simulink model "model_cnn"  (R2020a)
settings: Solver=VariableStepAuto  StartTime=0.0  StopTime=1e6/fs  RelTol=1e-3
PreLoadFcn:
  | setup_imports;
  | %dense2_numerictype = fixdt(1,18,10);
  | %conv1_numerictype = fixdt(1,18,21);
InitFcn:
  | % Intermediate signal dimensions
  | input_dim = [1, 2, 128];
  | layer1_dim = hInterConvLayerDims([1,3,1,64],input_dim,1); % dims : [C,H,W]
  | layer2_dim = hInterConvLayerDims([2,3,64,16],layer1_dim,1);% dims : [C,H,W]
  | layer3_dim = [1,128];
  | 
  | % Conv Layer 1 dimensions
  | conv1_dims = struct(...
  |     'input_dim',    input_dim,...       input_dim = C,H,W
  |     'filter_dim',   [1, 3, 1, 64],...  filter_dim = K,J,C,N
  |     'stride',       1,...
  |     'row_output',   3,...
  |     'output_dim',   layer1_dim);
  | 
  | % Conv Layer 2 dimensions
  | conv2_dims = struct(...
  |     'input_dim',    layer1_dim,...      input = C,H.W
  |     'filter_dim',   [2, 3, 64, 16],...  filter_dim = K,J,C,N
  |     'stride',       1,...
  |     'row_output',   2*3*64,...
  |     'output_dim',   layer2_dim);
  | 
  | % Dense Layer 1 dimensions
  | dense1_dims = struct(...
  |     'input_dim',    layer2_dim,...      input = C,H,W
  |     'weight_dim',   [1984, 128],...     weight_dim = H,W
  |     'output_dim',   layer3_dim);
  | 
  | % Load saved weights and input
  | setup_imports;
  | 
  | fs = 128e6;
  | fs_axi = 100e6;
  | R = 32;
values from neighbouring files (symbols this model uses):
  datatypeInput = X_test.numerictype    [setup_imports.m]
  gemm_wconv1 = fi(hInterleaveFilters(Wconv1),1,16)    [setup_imports.m]
  gemm_wconv2 = fi(hInterleaveFilters(Wconv2),1,16)    [setup_imports.m]
  wdense1 = fi(Wdense1,1,16)    [setup_imports.m]
  wdense2 = fi(Wdense2,1,16)    [setup_imports.m]
undefined symbols (not defined in the file or in its folder): ltehdlRAMinitPO2
libraries: hdlsllib x1022, dspsigops x3, dspsrcs4 x2
(part 11 of 23)

== system model_cnn/HDL CNN Model/Dense Layer 1/Dense Layer 1/adder50 ==
  In1 : Inport
  In2 : Inport  Port=2
  In3 : Inport  Port=3
  Data Type Conversion : DataTypeConversion  OutDataTypeStr=datatypeLayer3
  Multiply-Accumulate : hdlsllib/HDL Operations/Multiply-Accumulate  opMode=Streaming - using Number of Samples  initValueSetting=Dialog  initValue=0  initValueSetting2=Dialog  initValue2=0  initValueSetting3=Dialog  initValue3=0  num_samples=1984  RndMeth2=Floor  RndMeth3=Floor  datatype2=Inherit: Inherit via back propagation  datatype3=accumoutdatatype3  validOut=on  endInandOut=on  startOut=on  countOut=on  dim=-1  DoSatur=off  parallel=off
      settings: SourceProductBaseCode=SL
  Terminator : Terminator
  Terminator1 : Terminator
  Terminator2 : Terminator
  dataOut : Outport
  wires:
  Data Type Conversion/1 -> dataOut/1
  ? -> Terminator1/1  "validOut"
  In2/1 -> Multiply-Accumulate/1
  In3/1 -> ?
  Multiply-Accumulate/1 -> Data Type Conversion/1
  ? -> Terminator/1  "countOut"
  In1/1 -> Multiply-Accumulate/2
  ? -> Terminator2/1  "vectorOutValid"

== system model_cnn/HDL CNN Model/Dense Layer 1/Dense Layer 1/adder51 ==
  In1 : Inport
  In2 : Inport  Port=2
  In3 : Inport  Port=3
  Data Type Conversion : DataTypeConversion  OutDataTypeStr=datatypeLayer3
  Multiply-Accumulate : hdlsllib/HDL Operations/Multiply-Accumulate  opMode=Streaming - using Number of Samples  initValueSetting=Dialog  initValue=0  initValueSetting2=Dialog  initValue2=0  initValueSetting3=Dialog  initValue3=0  num_samples=1984  RndMeth2=Floor  RndMeth3=Floor  datatype2=Inherit: Inherit via back propagation  datatype3=accumoutdatatype3  validOut=on  endInandOut=on  startOut=on  countOut=on  dim=-1  DoSatur=off  parallel=off
      settings: SourceProductBaseCode=SL
  Terminator : Terminator
  Terminator1 : Terminator
  Terminator2 : Terminator
  dataOut : Outport
  wires:
  Data Type Conversion/1 -> dataOut/1
  ? -> Terminator1/1  "validOut"
  In2/1 -> Multiply-Accumulate/1
  In3/1 -> ?
  Multiply-Accumulate/1 -> Data Type Conversion/1
  ? -> Terminator/1  "countOut"
  In1/1 -> Multiply-Accumulate/2
  ? -> Terminator2/1  "vectorOutValid"

== system model_cnn/HDL CNN Model/Dense Layer 1/Dense Layer 1/adder52 ==
  In1 : Inport
  In2 : Inport  Port=2
  In3 : Inport  Port=3
  Data Type Conversion : DataTypeConversion  OutDataTypeStr=datatypeLayer3
  Multiply-Accumulate : hdlsllib/HDL Operations/Multiply-Accumulate  opMode=Streaming - using Number of Samples  initValueSetting=Dialog  initValue=0  initValueSetting2=Dialog  initValue2=0  initValueSetting3=Dialog  initValue3=0  num_samples=1984  RndMeth2=Floor  RndMeth3=Floor  datatype2=Inherit: Inherit via back propagation  datatype3=accumoutdatatype3  validOut=on  endInandOut=on  startOut=on  countOut=on  dim=-1  DoSatur=off  parallel=off
      settings: SourceProductBaseCode=SL
  Terminator : Terminator
  Terminator1 : Terminator
  Terminator2 : Terminator
  dataOut : Outport
  wires:
  Data Type Conversion/1 -> dataOut/1
  ? -> Terminator1/1  "validOut"
  In2/1 -> Multiply-Accumulate/1
  In3/1 -> ?
  Multiply-Accumulate/1 -> Data Type Conversion/1
  ? -> Terminator/1  "countOut"
  In1/1 -> Multiply-Accumulate/2
  ? -> Terminator2/1  "vectorOutValid"

== system model_cnn/HDL CNN Model/Dense Layer 1/Dense Layer 1/adder53 ==
  In1 : Inport
  In2 : Inport  Port=2
  In3 : Inport  Port=3
  Data Type Conversion : DataTypeConversion  OutDataTypeStr=datatypeLayer3
  Multiply-Accumulate : hdlsllib/HDL Operations/Multiply-Accumulate  opMode=Streaming - using Number of Samples  initValueSetting=Dialog  initValue=0  initValueSetting2=Dialog  initValue2=0  initValueSetting3=Dialog  initValue3=0  num_samples=1984  RndMeth2=Floor  RndMeth3=Floor  datatype2=Inherit: Inherit via back propagation  datatype3=accumoutdatatype3  validOut=on  endInandOut=on  startOut=on  countOut=on  dim=-1  DoSatur=off  parallel=off
      settings: SourceProductBaseCode=SL
  Terminator : Terminator
  Terminator1 : Terminator
  Terminator2 : Terminator
  dataOut : Outport
  wires:
  Data Type Conversion/1 -> dataOut/1
  ? -> Terminator1/1  "validOut"
  In2/1 -> Multiply-Accumulate/1
  In3/1 -> ?
  Multiply-Accumulate/1 -> Data Type Conversion/1
  ? -> Terminator/1  "countOut"
  In1/1 -> Multiply-Accumulate/2
  ? -> Terminator2/1  "vectorOutValid"

== system model_cnn/HDL CNN Model/Dense Layer 1/Dense Layer 1/adder54 ==
  In1 : Inport
  In2 : Inport  Port=2
  In3 : Inport  Port=3
  Data Type Conversion : DataTypeConversion  OutDataTypeStr=datatypeLayer3
  Multiply-Accumulate : hdlsllib/HDL Operations/Multiply-Accumulate  opMode=Streaming - using Number of Samples  initValueSetting=Dialog  initValue=0  initValueSetting2=Dialog  initValue2=0  initValueSetting3=Dialog  initValue3=0  num_samples=1984  RndMeth2=Floor  RndMeth3=Floor  datatype2=Inherit: Inherit via back propagation  datatype3=accumoutdatatype3  validOut=on  endInandOut=on  startOut=on  countOut=on  dim=-1  DoSatur=off  parallel=off
      settings: SourceProductBaseCode=SL
  Terminator : Terminator
  Terminator1 : Terminator
  Terminator2 : Terminator
  dataOut : Outport
  wires:
  Data Type Conversion/1 -> dataOut/1
  ? -> Terminator1/1  "validOut"
  In2/1 -> Multiply-Accumulate/1
  In3/1 -> ?
  Multiply-Accumulate/1 -> Data Type Conversion/1
  ? -> Terminator/1  "countOut"
  In1/1 -> Multiply-Accumulate/2
  ? -> Terminator2/1  "vectorOutValid"

== system model_cnn/HDL CNN Model/Dense Layer 1/Dense Layer 1/adder55 ==
  In1 : Inport
  In2 : Inport  Port=2
  In3 : Inport  Port=3
  Data Type Conversion : DataTypeConversion  OutDataTypeStr=datatypeLayer3
  Multiply-Accumulate : hdlsllib/HDL Operations/Multiply-Accumulate  opMode=Streaming - using Number of Samples  initValueSetting=Dialog  initValue=0  initValueSetting2=Dialog  initValue2=0  initValueSetting3=Dialog  initValue3=0  num_samples=1984  RndMeth2=Floor  RndMeth3=Floor  datatype2=Inherit: Inherit via back propagation  datatype3=accumoutdatatype3  validOut=on  endInandOut=on  startOut=on  countOut=on  dim=-1  DoSatur=off  parallel=off
      settings: SourceProductBaseCode=SL
  Terminator : Terminator
  Terminator1 : Terminator
  Terminator2 : Terminator
  dataOut : Outport
  wires:
  Data Type Conversion/1 -> dataOut/1
  ? -> Terminator1/1  "validOut"
  In2/1 -> Multiply-Accumulate/1
  In3/1 -> ?
  Multiply-Accumulate/1 -> Data Type Conversion/1
  ? -> Terminator/1  "countOut"
  In1/1 -> Multiply-Accumulate/2
  ? -> Terminator2/1  "vectorOutValid"

== system model_cnn/HDL CNN Model/Dense Layer 1/Dense Layer 1/adder56 ==
  In1 : Inport
  In2 : Inport  Port=2
  In3 : Inport  Port=3
  Data Type Conversion : DataTypeConversion  OutDataTypeStr=datatypeLayer3
  Multiply-Accumulate : hdlsllib/HDL Operations/Multiply-Accumulate  opMode=Streaming - using Number of Samples  initValueSetting=Dialog  initValue=0  initValueSetting2=Dialog  initValue2=0  initValueSetting3=Dialog  initValue3=0  num_samples=1984  RndMeth2=Floor  RndMeth3=Floor  datatype2=Inherit: Inherit via back propagation  datatype3=accumoutdatatype3  validOut=on  endInandOut=on  startOut=on  countOut=on  dim=-1  DoSatur=off  parallel=off
      settings: SourceProductBaseCode=SL
  Terminator : Terminator
  Terminator1 : Terminator
  Terminator2 : Terminator
  dataOut : Outport
  wires:
  Data Type Conversion/1 -> dataOut/1
  ? -> Terminator1/1  "validOut"
  In2/1 -> Multiply-Accumulate/1
  In3/1 -> ?
  Multiply-Accumulate/1 -> Data Type Conversion/1
  ? -> Terminator/1  "countOut"
  In1/1 -> Multiply-Accumulate/2
  ? -> Terminator2/1  "vectorOutValid"

== system model_cnn/HDL CNN Model/Dense Layer 1/Dense Layer 1/adder57 ==
  In1 : Inport
  In2 : Inport  Port=2
  In3 : Inport  Port=3
  Data Type Conversion : DataTypeConversion  OutDataTypeStr=datatypeLayer3
  Multiply-Accumulate : hdlsllib/HDL Operations/Multiply-Accumulate  opMode=Streaming - using Number of Samples  initValueSetting=Dialog  initValue=0  initValueSetting2=Dialog  initValue2=0  initValueSetting3=Dialog  initValue3=0  num_samples=1984  RndMeth2=Floor  RndMeth3=Floor  datatype2=Inherit: Inherit via back propagation  datatype3=accumoutdatatype3  validOut=on  endInandOut=on  startOut=on  countOut=on  dim=-1  DoSatur=off  parallel=off
      settings: SourceProductBaseCode=SL
  Terminator : Terminator
  Terminator1 : Terminator
  Terminator2 : Terminator
  dataOut : Outport
  wires:
  Data Type Conversion/1 -> dataOut/1
  ? -> Terminator1/1  "validOut"
  In2/1 -> Multiply-Accumulate/1
  In3/1 -> ?
  Multiply-Accumulate/1 -> Data Type Conversion/1
  ? -> Terminator/1  "countOut"
  In1/1 -> Multiply-Accumulate/2
  ? -> Terminator2/1  "vectorOutValid"

== system model_cnn/HDL CNN Model/Dense Layer 1/Dense Layer 1/adder58 ==
  In1 : Inport
  In2 : Inport  Port=2
  In3 : Inport  Port=3
  Data Type Conversion : DataTypeConversion  OutDataTypeStr=datatypeLayer3
  Multiply-Accumulate : hdlsllib/HDL Operations/Multiply-Accumulate  opMode=Streaming - using Number of Samples  initValueSetting=Dialog  initValue=0  initValueSetting2=Dialog  initValue2=0  initValueSetting3=Dialog  initValue3=0  num_samples=1984  RndMeth2=Floor  RndMeth3=Floor  datatype2=Inherit: Inherit via back propagation  datatype3=accumoutdatatype3  validOut=on  endInandOut=on  startOut=on  countOut=on  dim=-1  DoSatur=off  parallel=off
      settings: SourceProductBaseCode=SL
  Terminator : Terminator
  Terminator1 : Terminator
  Terminator2 : Terminator
  dataOut : Outport
  wires:
  Data Type Conversion/1 -> dataOut/1
  ? -> Terminator1/1  "validOut"
  In2/1 -> Multiply-Accumulate/1
  In3/1 -> ?
  Multiply-Accumulate/1 -> Data Type Conversion/1
  ? -> Terminator/1  "countOut"
  In1/1 -> Multiply-Accumulate/2
  ? -> Terminator2/1  "vectorOutValid"

== system model_cnn/HDL CNN Model/Dense Layer 1/Dense Layer 1/adder59 ==
  In1 : Inport
  In2 : Inport  Port=2
  In3 : Inport  Port=3
  Data Type Conversion : DataTypeConversion  OutDataTypeStr=datatypeLayer3
  Multiply-Accumulate : hdlsllib/HDL Operations/Multiply-Accumulate  opMode=Streaming - using Number of Samples  initValueSetting=Dialog  initValue=0  initValueSetting2=Dialog  initValue2=0  initValueSetting3=Dialog  initValue3=0  num_samples=1984  RndMeth2=Floor  RndMeth3=Floor  datatype2=Inherit: Inherit via back propagation  datatype3=accumoutdatatype3  validOut=on  endInandOut=on  startOut=on  countOut=on  dim=-1  DoSatur=off  parallel=off
      settings: SourceProductBaseCode=SL
  Terminator : Terminator
  Terminator1 : Terminator
  Terminator2 : Terminator
  dataOut : Outport
  wires:
  Data Type Conversion/1 -> dataOut/1
  ? -> Terminator1/1  "validOut"
  In2/1 -> Multiply-Accumulate/1
  In3/1 -> ?
  Multiply-Accumulate/1 -> Data Type Conversion/1
  ? -> Terminator/1  "countOut"
  In1/1 -> Multiply-Accumulate/2
  ? -> Terminator2/1  "vectorOutValid"

== system model_cnn/HDL CNN Model/Dense Layer 1/Dense Layer 1/adder6 ==
  In1 : Inport
  In2 : Inport  Port=2
  In3 : Inport  Port=3
  Data Type Conversion : DataTypeConversion  OutDataTypeStr=datatypeLayer3
  Multiply-Accumulate : hdlsllib/HDL Operations/Multiply-Accumulate  opMode=Streaming - using Number of Samples  initValueSetting=Dialog  initValue=0  initValueSetting2=Dialog  initValue2=0  initValueSetting3=Dialog  initValue3=0  num_samples=1984  RndMeth2=Floor  RndMeth3=Floor  datatype2=Inherit: Inherit via back propagation  datatype3=accumoutdatatype3  validOut=on  endInandOut=on  startOut=on  countOut=on  dim=-1  DoSatur=off  parallel=off
      settings: SourceProductBaseCode=SL
  Terminator : Terminator
  Terminator1 : Terminator
  Terminator2 : Terminator
  dataOut : Outport
  wires:
  Data Type Conversion/1 -> dataOut/1
  ? -> Terminator1/1  "validOut"
  In2/1 -> Multiply-Accumulate/1
  In3/1 -> ?
  Multiply-Accumulate/1 -> Data Type Conversion/1
  ? -> Terminator/1  "countOut"
  In1/1 -> Multiply-Accumulate/2
  ? -> Terminator2/1  "vectorOutValid"

== system model_cnn/HDL CNN Model/Dense Layer 1/Dense Layer 1/adder60 ==
  In1 : Inport
  In2 : Inport  Port=2
  In3 : Inport  Port=3
  Data Type Conversion : DataTypeConversion  OutDataTypeStr=datatypeLayer3
  Multiply-Accumulate : hdlsllib/HDL Operations/Multiply-Accumulate  opMode=Streaming - using Number of Samples  initValueSetting=Dialog  initValue=0  initValueSetting2=Dialog  initValue2=0  initValueSetting3=Dialog  initValue3=0  num_samples=1984  RndMeth2=Floor  RndMeth3=Floor  datatype2=Inherit: Inherit via back propagation  datatype3=accumoutdatatype3  validOut=on  endInandOut=on  startOut=on  countOut=on  dim=-1  DoSatur=off  parallel=off
      settings: SourceProductBaseCode=SL
  Terminator : Terminator
  Terminator1 : Terminator
  Terminator2 : Terminator
  dataOut : Outport
  wires:
  Data Type Conversion/1 -> dataOut/1
  ? -> Terminator1/1  "validOut"
  In2/1 -> Multiply-Accumulate/1
  In3/1 -> ?
  Multiply-Accumulate/1 -> Data Type Conversion/1
  ? -> Terminator/1  "countOut"
  In1/1 -> Multiply-Accumulate/2
  ? -> Terminator2/1  "vectorOutValid"

== system model_cnn/HDL CNN Model/Dense Layer 1/Dense Layer 1/adder61 ==
  In1 : Inport
  In2 : Inport  Port=2
  In3 : Inport  Port=3
  Data Type Conversion : DataTypeConversion  OutDataTypeStr=datatypeLayer3
  Multiply-Accumulate : hdlsllib/HDL Operations/Multiply-Accumulate  opMode=Streaming - using Number of Samples  initValueSetting=Dialog  initValue=0  initValueSetting2=Dialog  initValue2=0  initValueSetting3=Dialog  initValue3=0  num_samples=1984  RndMeth2=Floor  RndMeth3=Floor  datatype2=Inherit: Inherit via back propagation  datatype3=accumoutdatatype3  validOut=on  endInandOut=on  startOut=on  countOut=on  dim=-1  DoSatur=off  parallel=off
      settings: SourceProductBaseCode=SL
  Terminator : Terminator
  Terminator1 : Terminator
  Terminator2 : Terminator
  dataOut : Outport
  wires:
  Data Type Conversion/1 -> dataOut/1
  ? -> Terminator1/1  "validOut"
  In2/1 -> Multiply-Accumulate/1
  In3/1 -> ?
  Multiply-Accumulate/1 -> Data Type Conversion/1
  ? -> Terminator/1  "countOut"
  In1/1 -> Multiply-Accumulate/2
  ? -> Terminator2/1  "vectorOutValid"

== system model_cnn/HDL CNN Model/Dense Layer 1/Dense Layer 1/adder62 ==
  In1 : Inport
  In2 : Inport  Port=2
  In3 : Inport  Port=3
  Data Type Conversion : DataTypeConversion  OutDataTypeStr=datatypeLayer3
  Multiply-Accumulate : hdlsllib/HDL Operations/Multiply-Accumulate  opMode=Streaming - using Number of Samples  initValueSetting=Dialog  initValue=0  initValueSetting2=Dialog  initValue2=0  initValueSetting3=Dialog  initValue3=0  num_samples=1984  RndMeth2=Floor  RndMeth3=Floor  datatype2=Inherit: Inherit via back propagation  datatype3=accumoutdatatype3  validOut=on  endInandOut=on  startOut=on  countOut=on  dim=-1  DoSatur=off  parallel=off
      settings: SourceProductBaseCode=SL
  Terminator : Terminator
  Terminator1 : Terminator
  Terminator2 : Terminator
  dataOut : Outport
  wires:
  Data Type Conversion/1 -> dataOut/1
  ? -> Terminator1/1  "validOut"
  In2/1 -> Multiply-Accumulate/1
  In3/1 -> ?
  Multiply-Accumulate/1 -> Data Type Conversion/1
  ? -> Terminator/1  "countOut"
  In1/1 -> Multiply-Accumulate/2
  ? -> Terminator2/1  "vectorOutValid"

== system model_cnn/HDL CNN Model/Dense Layer 1/Dense Layer 1/adder63 ==
  In1 : Inport
  In2 : Inport  Port=2
  In3 : Inport  Port=3
  Data Type Conversion : DataTypeConversion  OutDataTypeStr=datatypeLayer3
  Multiply-Accumulate : hdlsllib/HDL Operations/Multiply-Accumulate  opMode=Streaming - using Number of Samples  initValueSetting=Dialog  initValue=0  initValueSetting2=Dialog  initValue2=0  initValueSetting3=Dialog  initValue3=0  num_samples=1984  RndMeth2=Floor  RndMeth3=Floor  datatype2=Inherit: Inherit via back propagation  datatype3=accumoutdatatype3  validOut=on  endInandOut=on  startOut=on  countOut=on  dim=-1  DoSatur=off  parallel=off
      settings: SourceProductBaseCode=SL
  Terminator : Terminator
  Terminator1 : Terminator
  Terminator2 : Terminator
  dataOut : Outport
  wires:
  Data Type Conversion/1 -> dataOut/1
  ? -> Terminator1/1  "validOut"
  In2/1 -> Multiply-Accumulate/1
  In3/1 -> ?
  Multiply-Accumulate/1 -> Data Type Conversion/1
  ? -> Terminator/1  "countOut"
  In1/1 -> Multiply-Accumulate/2
  ? -> Terminator2/1  "vectorOutValid"

== system model_cnn/HDL CNN Model/Dense Layer 1/Dense Layer 1/adder64 ==
  In1 : Inport
  In2 : Inport  Port=2
  In3 : Inport  Port=3
  Data Type Conversion : DataTypeConversion  OutDataTypeStr=datatypeLayer3
  Multiply-Accumulate : hdlsllib/HDL Operations/Multiply-Accumulate  opMode=Streaming - using Number of Samples  initValueSetting=Dialog  initValue=0  initValueSetting2=Dialog  initValue2=0  initValueSetting3=Dialog  initValue3=0  num_samples=1984  RndMeth2=Floor  RndMeth3=Floor  datatype2=Inherit: Inherit via back propagation  datatype3=accumoutdatatype3  validOut=on  endInandOut=on  startOut=on  countOut=on  dim=-1  DoSatur=off  parallel=off
      settings: SourceProductBaseCode=SL
  Terminator : Terminator
  Terminator1 : Terminator
  Terminator2 : Terminator
  dataOut : Outport
  wires:
  Data Type Conversion/1 -> dataOut/1
  ? -> Terminator1/1  "validOut"
  In2/1 -> Multiply-Accumulate/1
  In3/1 -> ?
  Multiply-Accumulate/1 -> Data Type Conversion/1
  ? -> Terminator/1  "countOut"
  In1/1 -> Multiply-Accumulate/2
  ? -> Terminator2/1  "vectorOutValid"

== system model_cnn/HDL CNN Model/Dense Layer 1/Dense Layer 1/adder65 ==
  In1 : Inport
  In2 : Inport  Port=2
  In3 : Inport  Port=3
  Data Type Conversion : DataTypeConversion  OutDataTypeStr=datatypeLayer3
  Multiply-Accumulate : hdlsllib/HDL Operations/Multiply-Accumulate  opMode=Streaming - using Number of Samples  initValueSetting=Dialog  initValue=0  initValueSetting2=Dialog  initValue2=0  initValueSetting3=Dialog  initValue3=0  num_samples=1984  RndMeth2=Floor  RndMeth3=Floor  datatype2=Inherit: Inherit via back propagation  datatype3=accumoutdatatype3  validOut=on  endInandOut=on  startOut=on  countOut=on  dim=-1  DoSatur=off  parallel=off
      settings: SourceProductBaseCode=SL
  Terminator : Terminator
  Terminator1 : Terminator
  Terminator2 : Terminator
  dataOut : Outport
  wires:
  Data Type Conversion/1 -> dataOut/1
  ? -> Terminator1/1  "validOut"
  In2/1 -> Multiply-Accumulate/1
  In3/1 -> ?
  Multiply-Accumulate/1 -> Data Type Conversion/1
  ? -> Terminator/1  "countOut"
  In1/1 -> Multiply-Accumulate/2
  ? -> Terminator2/1  "vectorOutValid"

== system model_cnn/HDL CNN Model/Dense Layer 1/Dense Layer 1/adder66 ==
  In1 : Inport
  In2 : Inport  Port=2
  In3 : Inport  Port=3
  Data Type Conversion : DataTypeConversion  OutDataTypeStr=datatypeLayer3
  Multiply-Accumulate : hdlsllib/HDL Operations/Multiply-Accumulate  opMode=Streaming - using Number of Samples  initValueSetting=Dialog  initValue=0  initValueSetting2=Dialog  initValue2=0  initValueSetting3=Dialog  initValue3=0  num_samples=1984  RndMeth2=Floor  RndMeth3=Floor  datatype2=Inherit: Inherit via back propagation  datatype3=accumoutdatatype3  validOut=on  endInandOut=on  startOut=on  countOut=on  dim=-1  DoSatur=off  parallel=off
      settings: SourceProductBaseCode=SL
  Terminator : Terminator
  Terminator1 : Terminator
  Terminator2 : Terminator
  dataOut : Outport
  wires:
  Data Type Conversion/1 -> dataOut/1
  ? -> Terminator1/1  "validOut"
  In2/1 -> Multiply-Accumulate/1
  In3/1 -> ?
  Multiply-Accumulate/1 -> Data Type Conversion/1
  ? -> Terminator/1  "countOut"
  In1/1 -> Multiply-Accumulate/2
  ? -> Terminator2/1  "vectorOutValid"

== system model_cnn/HDL CNN Model/Dense Layer 1/Dense Layer 1/adder67 ==
  In1 : Inport
  In2 : Inport  Port=2
  In3 : Inport  Port=3
  Data Type Conversion : DataTypeConversion  OutDataTypeStr=datatypeLayer3
  Multiply-Accumulate : hdlsllib/HDL Operations/Multiply-Accumulate  opMode=Streaming - using Number of Samples  initValueSetting=Dialog  initValue=0  initValueSetting2=Dialog  initValue2=0  initValueSetting3=Dialog  initValue3=0  num_samples=1984  RndMeth2=Floor  RndMeth3=Floor  datatype2=Inherit: Inherit via back propagation  datatype3=accumoutdatatype3  validOut=on  endInandOut=on  startOut=on  countOut=on  dim=-1  DoSatur=off  parallel=off
      settings: SourceProductBaseCode=SL
  Terminator : Terminator
  Terminator1 : Terminator
  Terminator2 : Terminator
  dataOut : Outport
  wires:
  Data Type Conversion/1 -> dataOut/1
  ? -> Terminator1/1  "validOut"
  In2/1 -> Multiply-Accumulate/1
  In3/1 -> ?
  Multiply-Accumulate/1 -> Data Type Conversion/1
  ? -> Terminator/1  "countOut"
  In1/1 -> Multiply-Accumulate/2
  ? -> Terminator2/1  "vectorOutValid"

== system model_cnn/HDL CNN Model/Dense Layer 1/Dense Layer 1/adder68 ==
  In1 : Inport
  In2 : Inport  Port=2
  In3 : Inport  Port=3
  Data Type Conversion : DataTypeConversion  OutDataTypeStr=datatypeLayer3
  Multiply-Accumulate : hdlsllib/HDL Operations/Multiply-Accumulate  opMode=Streaming - using Number of Samples  initValueSetting=Dialog  initValue=0  initValueSetting2=Dialog  initValue2=0  initValueSetting3=Dialog  initValue3=0  num_samples=1984  RndMeth2=Floor  RndMeth3=Floor  datatype2=Inherit: Inherit via back propagation  datatype3=accumoutdatatype3  validOut=on  endInandOut=on  startOut=on  countOut=on  dim=-1  DoSatur=off  parallel=off
      settings: SourceProductBaseCode=SL
  Terminator : Terminator
  Terminator1 : Terminator
  Terminator2 : Terminator
  dataOut : Outport
  wires:
  Data Type Conversion/1 -> dataOut/1
  ? -> Terminator1/1  "validOut"
  In2/1 -> Multiply-Accumulate/1
  In3/1 -> ?
  Multiply-Accumulate/1 -> Data Type Conversion/1
  ? -> Terminator/1  "countOut"
  In1/1 -> Multiply-Accumulate/2
  ? -> Terminator2/1  "vectorOutValid"

== system model_cnn/HDL CNN Model/Dense Layer 1/Dense Layer 1/adder69 ==
  In1 : Inport
  In2 : Inport  Port=2
  In3 : Inport  Port=3
  Data Type Conversion : DataTypeConversion  OutDataTypeStr=datatypeLayer3
  Multiply-Accumulate : hdlsllib/HDL Operations/Multiply-Accumulate  opMode=Streaming - using Number of Samples  initValueSetting=Dialog  initValue=0  initValueSetting2=Dialog  initValue2=0  initValueSetting3=Dialog  initValue3=0  num_samples=1984  RndMeth2=Floor  RndMeth3=Floor  datatype2=Inherit: Inherit via back propagation  datatype3=accumoutdatatype3  validOut=on  endInandOut=on  startOut=on  countOut=on  dim=-1  DoSatur=off  parallel=off
      settings: SourceProductBaseCode=SL
  Terminator : Terminator
  Terminator1 : Terminator
  Terminator2 : Terminator
  dataOut : Outport
  wires:
  Data Type Conversion/1 -> dataOut/1
  ? -> Terminator1/1  "validOut"
  In2/1 -> Multiply-Accumulate/1
  In3/1 -> ?
  Multiply-Accumulate/1 -> Data Type Conversion/1
  ? -> Terminator/1  "countOut"
  In1/1 -> Multiply-Accumulate/2
  ? -> Terminator2/1  "vectorOutValid"

== system model_cnn/HDL CNN Model/Dense Layer 1/Dense Layer 1/adder7 ==
  In1 : Inport
  In2 : Inport  Port=2
  In3 : Inport  Port=3
  Data Type Conversion : DataTypeConversion  OutDataTypeStr=datatypeLayer3
  Multiply-Accumulate : hdlsllib/HDL Operations/Multiply-Accumulate  opMode=Streaming - using Number of Samples  initValueSetting=Dialog  initValue=0  initValueSetting2=Dialog  initValue2=0  initValueSetting3=Dialog  initValue3=0  num_samples=1984  RndMeth2=Floor  RndMeth3=Floor  datatype2=Inherit: Inherit via back propagation  datatype3=accumoutdatatype3  validOut=on  endInandOut=on  startOut=on  countOut=on  dim=-1  DoSatur=off  parallel=off
      settings: SourceProductBaseCode=SL
  Terminator : Terminator
  Terminator1 : Terminator
  Terminator2 : Terminator
  dataOut : Outport
  wires:
  Data Type Conversion/1 -> dataOut/1
  ? -> Terminator1/1  "validOut"
  In2/1 -> Multiply-Accumulate/1
  In3/1 -> ?
  Multiply-Accumulate/1 -> Data Type Conversion/1
  ? -> Terminator/1  "countOut"
  In1/1 -> Multiply-Accumulate/2
  ? -> Terminator2/1  "vectorOutValid"

== system model_cnn/HDL CNN Model/Dense Layer 1/Dense Layer 1/adder70 ==
  In1 : Inport
  In2 : Inport  Port=2
  In3 : Inport  Port=3
  Data Type Conversion : DataTypeConversion  OutDataTypeStr=datatypeLayer3
  Multiply-Accumulate : hdlsllib/HDL Operations/Multiply-Accumulate  opMode=Streaming - using Number of Samples  initValueSetting=Dialog  initValue=0  initValueSetting2=Dialog  initValue2=0  initValueSetting3=Dialog  initValue3=0  num_samples=1984  RndMeth2=Floor  RndMeth3=Floor  datatype2=Inherit: Inherit via back propagation  datatype3=accumoutdatatype3  validOut=on  endInandOut=on  startOut=on  countOut=on  dim=-1  DoSatur=off  parallel=off
      settings: SourceProductBaseCode=SL
  Terminator : Terminator
  Terminator1 : Terminator
  Terminator2 : Terminator
  dataOut : Outport
  wires:
  Data Type Conversion/1 -> dataOut/1
  ? -> Terminator1/1  "validOut"
  In2/1 -> Multiply-Accumulate/1
  In3/1 -> ?
  Multiply-Accumulate/1 -> Data Type Conversion/1
  ? -> Terminator/1  "countOut"
  In1/1 -> Multiply-Accumulate/2
  ? -> Terminator2/1  "vectorOutValid"

== system model_cnn/HDL CNN Model/Dense Layer 1/Dense Layer 1/adder71 ==
  In1 : Inport
  In2 : Inport  Port=2
  In3 : Inport  Port=3
  Data Type Conversion : DataTypeConversion  OutDataTypeStr=datatypeLayer3
  Multiply-Accumulate : hdlsllib/HDL Operations/Multiply-Accumulate  opMode=Streaming - using Number of Samples  initValueSetting=Dialog  initValue=0  initValueSetting2=Dialog  initValue2=0  initValueSetting3=Dialog  initValue3=0  num_samples=1984  RndMeth2=Floor  RndMeth3=Floor  datatype2=Inherit: Inherit via back propagation  datatype3=accumoutdatatype3  validOut=on  endInandOut=on  startOut=on  countOut=on  dim=-1  DoSatur=off  parallel=off
      settings: SourceProductBaseCode=SL
  Terminator : Terminator
  Terminator1 : Terminator
  Terminator2 : Terminator
  dataOut : Outport
  wires:
  Data Type Conversion/1 -> dataOut/1
  ? -> Terminator1/1  "validOut"
  In2/1 -> Multiply-Accumulate/1
  In3/1 -> ?
  Multiply-Accumulate/1 -> Data Type Conversion/1
  ? -> Terminator/1  "countOut"
  In1/1 -> Multiply-Accumulate/2
  ? -> Terminator2/1  "vectorOutValid"

== system model_cnn/HDL CNN Model/Dense Layer 1/Dense Layer 1/adder72 ==
  In1 : Inport
  In2 : Inport  Port=2
  In3 : Inport  Port=3
  Data Type Conversion : DataTypeConversion  OutDataTypeStr=datatypeLayer3
  Multiply-Accumulate : hdlsllib/HDL Operations/Multiply-Accumulate  opMode=Streaming - using Number of Samples  initValueSetting=Dialog  initValue=0  initValueSetting2=Dialog  initValue2=0  initValueSetting3=Dialog  initValue3=0  num_samples=1984  RndMeth2=Floor  RndMeth3=Floor  datatype2=Inherit: Inherit via back propagation  datatype3=accumoutdatatype3  validOut=on  endInandOut=on  startOut=on  countOut=on  dim=-1  DoSatur=off  parallel=off
      settings: SourceProductBaseCode=SL
  Terminator : Terminator
  Terminator1 : Terminator
  Terminator2 : Terminator
  dataOut : Outport
  wires:
  Data Type Conversion/1 -> dataOut/1
  ? -> Terminator1/1  "validOut"
  In2/1 -> Multiply-Accumulate/1
  In3/1 -> ?
  Multiply-Accumulate/1 -> Data Type Conversion/1
  ? -> Terminator/1  "countOut"
  In1/1 -> Multiply-Accumulate/2
  ? -> Terminator2/1  "vectorOutValid"

== system model_cnn/HDL CNN Model/Dense Layer 1/Dense Layer 1/adder73 ==
  In1 : Inport
  In2 : Inport  Port=2
  In3 : Inport  Port=3
  Data Type Conversion : DataTypeConversion  OutDataTypeStr=datatypeLayer3
  Multiply-Accumulate : hdlsllib/HDL Operations/Multiply-Accumulate  opMode=Streaming - using Number of Samples  initValueSetting=Dialog  initValue=0  initValueSetting2=Dialog  initValue2=0  initValueSetting3=Dialog  initValue3=0  num_samples=1984  RndMeth2=Floor  RndMeth3=Floor  datatype2=Inherit: Inherit via back propagation  datatype3=accumoutdatatype3  validOut=on  endInandOut=on  startOut=on  countOut=on  dim=-1  DoSatur=off  parallel=off
      settings: SourceProductBaseCode=SL
  Terminator : Terminator
  Terminator1 : Terminator
  Terminator2 : Terminator
  dataOut : Outport
  wires:
  Data Type Conversion/1 -> dataOut/1
  ? -> Terminator1/1  "validOut"
  In2/1 -> Multiply-Accumulate/1
  In3/1 -> ?
  Multiply-Accumulate/1 -> Data Type Conversion/1
  ? -> Terminator/1  "countOut"
  In1/1 -> Multiply-Accumulate/2
  ? -> Terminator2/1  "vectorOutValid"

== system model_cnn/HDL CNN Model/Dense Layer 1/Dense Layer 1/adder74 ==
  In1 : Inport
  In2 : Inport  Port=2
  In3 : Inport  Port=3
  Data Type Conversion : DataTypeConversion  OutDataTypeStr=datatypeLayer3
  Multiply-Accumulate : hdlsllib/HDL Operations/Multiply-Accumulate  opMode=Streaming - using Number of Samples  initValueSetting=Dialog  initValue=0  initValueSetting2=Dialog  initValue2=0  initValueSetting3=Dialog  initValue3=0  num_samples=1984  RndMeth2=Floor  RndMeth3=Floor  datatype2=Inherit: Inherit via back propagation  datatype3=accumoutdatatype3  validOut=on  endInandOut=on  startOut=on  countOut=on  dim=-1  DoSatur=off  parallel=off
      settings: SourceProductBaseCode=SL
  Terminator : Terminator
  Terminator1 : Terminator
  Terminator2 : Terminator
  dataOut : Outport
  wires:
  Data Type Conversion/1 -> dataOut/1
  ? -> Terminator1/1  "validOut"
  In2/1 -> Multiply-Accumulate/1
  In3/1 -> ?
  Multiply-Accumulate/1 -> Data Type Conversion/1
  ? -> Terminator/1  "countOut"
  In1/1 -> Multiply-Accumulate/2
  ? -> Terminator2/1  "vectorOutValid"

== system model_cnn/HDL CNN Model/Dense Layer 1/Dense Layer 1/adder75 ==
  In1 : Inport
  In2 : Inport  Port=2
  In3 : Inport  Port=3
  Data Type Conversion : DataTypeConversion  OutDataTypeStr=datatypeLayer3
  Multiply-Accumulate : hdlsllib/HDL Operations/Multiply-Accumulate  opMode=Streaming - using Number of Samples  initValueSetting=Dialog  initValue=0  initValueSetting2=Dialog  initValue2=0  initValueSetting3=Dialog  initValue3=0  num_samples=1984  RndMeth2=Floor  RndMeth3=Floor  datatype2=Inherit: Inherit via back propagation  datatype3=accumoutdatatype3  validOut=on  endInandOut=on  startOut=on  countOut=on  dim=-1  DoSatur=off  parallel=off
      settings: SourceProductBaseCode=SL
  Terminator : Terminator
  Terminator1 : Terminator
  Terminator2 : Terminator
  dataOut : Outport
  wires:
  Data Type Conversion/1 -> dataOut/1
  ? -> Terminator1/1  "validOut"
  In2/1 -> Multiply-Accumulate/1
  In3/1 -> ?
  Multiply-Accumulate/1 -> Data Type Conversion/1
  ? -> Terminator/1  "countOut"
  In1/1 -> Multiply-Accumulate/2
  ? -> Terminator2/1  "vectorOutValid"

== system model_cnn/HDL CNN Model/Dense Layer 1/Dense Layer 1/adder76 ==
  In1 : Inport
  In2 : Inport  Port=2
  In3 : Inport  Port=3
  Data Type Conversion : DataTypeConversion  OutDataTypeStr=datatypeLayer3
  Multiply-Accumulate : hdlsllib/HDL Operations/Multiply-Accumulate  opMode=Streaming - using Number of Samples  initValueSetting=Dialog  initValue=0  initValueSetting2=Dialog  initValue2=0  initValueSetting3=Dialog  initValue3=0  num_samples=1984  RndMeth2=Floor  RndMeth3=Floor  datatype2=Inherit: Inherit via back propagation  datatype3=accumoutdatatype3  validOut=on  endInandOut=on  startOut=on  countOut=on  dim=-1  DoSatur=off  parallel=off
      settings: SourceProductBaseCode=SL
  Terminator : Terminator
  Terminator1 : Terminator
  Terminator2 : Terminator
  dataOut : Outport
  wires:
  Data Type Conversion/1 -> dataOut/1
  ? -> Terminator1/1  "validOut"
  In2/1 -> Multiply-Accumulate/1
  In3/1 -> ?
  Multiply-Accumulate/1 -> Data Type Conversion/1
  ? -> Terminator/1  "countOut"
  In1/1 -> Multiply-Accumulate/2
  ? -> Terminator2/1  "vectorOutValid"

== system model_cnn/HDL CNN Model/Dense Layer 1/Dense Layer 1/adder77 ==
  In1 : Inport
  In2 : Inport  Port=2
  In3 : Inport  Port=3
  Data Type Conversion : DataTypeConversion  OutDataTypeStr=datatypeLayer3
  Multiply-Accumulate : hdlsllib/HDL Operations/Multiply-Accumulate  opMode=Streaming - using Number of Samples  initValueSetting=Dialog  initValue=0  initValueSetting2=Dialog  initValue2=0  initValueSetting3=Dialog  initValue3=0  num_samples=1984  RndMeth2=Floor  RndMeth3=Floor  datatype2=Inherit: Inherit via back propagation  datatype3=accumoutdatatype3  validOut=on  endInandOut=on  startOut=on  countOut=on  dim=-1  DoSatur=off  parallel=off
      settings: SourceProductBaseCode=SL
  Terminator : Terminator
  Terminator1 : Terminator
  Terminator2 : Terminator
  dataOut : Outport
  wires:
  Data Type Conversion/1 -> dataOut/1
  ? -> Terminator1/1  "validOut"
  In2/1 -> Multiply-Accumulate/1
  In3/1 -> ?
  Multiply-Accumulate/1 -> Data Type Conversion/1
  ? -> Terminator/1  "countOut"
  In1/1 -> Multiply-Accumulate/2
  ? -> Terminator2/1  "vectorOutValid"

== system model_cnn/HDL CNN Model/Dense Layer 1/Dense Layer 1/adder78 ==
  In1 : Inport
  In2 : Inport  Port=2
  In3 : Inport  Port=3
  Data Type Conversion : DataTypeConversion  OutDataTypeStr=datatypeLayer3
  Multiply-Accumulate : hdlsllib/HDL Operations/Multiply-Accumulate  opMode=Streaming - using Number of Samples  initValueSetting=Dialog  initValue=0  initValueSetting2=Dialog  initValue2=0  initValueSetting3=Dialog  initValue3=0  num_samples=1984  RndMeth2=Floor  RndMeth3=Floor  datatype2=Inherit: Inherit via back propagation  datatype3=accumoutdatatype3  validOut=on  endInandOut=on  startOut=on  countOut=on  dim=-1  DoSatur=off  parallel=off
      settings: SourceProductBaseCode=SL
  Terminator : Terminator
  Terminator1 : Terminator
  Terminator2 : Terminator
  dataOut : Outport
  wires:
  Data Type Conversion/1 -> dataOut/1
  ? -> Terminator1/1  "validOut"
  In2/1 -> Multiply-Accumulate/1
  In3/1 -> ?
  Multiply-Accumulate/1 -> Data Type Conversion/1
  ? -> Terminator/1  "countOut"
  In1/1 -> Multiply-Accumulate/2
  ? -> Terminator2/1  "vectorOutValid"

== system model_cnn/HDL CNN Model/Dense Layer 1/Dense Layer 1/adder79 ==
  In1 : Inport
  In2 : Inport  Port=2
  In3 : Inport  Port=3
  Data Type Conversion : DataTypeConversion  OutDataTypeStr=datatypeLayer3
  Multiply-Accumulate : hdlsllib/HDL Operations/Multiply-Accumulate  opMode=Streaming - using Number of Samples  initValueSetting=Dialog  initValue=0  initValueSetting2=Dialog  initValue2=0  initValueSetting3=Dialog  initValue3=0  num_samples=1984  RndMeth2=Floor  RndMeth3=Floor  datatype2=Inherit: Inherit via back propagation  datatype3=accumoutdatatype3  validOut=on  endInandOut=on  startOut=on  countOut=on  dim=-1  DoSatur=off  parallel=off
      settings: SourceProductBaseCode=SL
  Terminator : Terminator
  Terminator1 : Terminator
  Terminator2 : Terminator
  dataOut : Outport
  wires:
  Data Type Conversion/1 -> dataOut/1
  ? -> Terminator1/1  "validOut"
  In2/1 -> Multiply-Accumulate/1
  In3/1 -> ?
  Multiply-Accumulate/1 -> Data Type Conversion/1
  ? -> Terminator/1  "countOut"
  In1/1 -> Multiply-Accumulate/2
  ? -> Terminator2/1  "vectorOutValid"

== system model_cnn/HDL CNN Model/Dense Layer 1/Dense Layer 1/adder8 ==
  In1 : Inport
  In2 : Inport  Port=2
  In3 : Inport  Port=3
  Data Type Conversion : DataTypeConversion  OutDataTypeStr=datatypeLayer3
  Multiply-Accumulate : hdlsllib/HDL Operations/Multiply-Accumulate  opMode=Streaming - using Number of Samples  initValueSetting=Dialog  initValue=0  initValueSetting2=Dialog  initValue2=0  initValueSetting3=Dialog  initValue3=0  num_samples=1984  RndMeth2=Floor  RndMeth3=Floor  datatype2=Inherit: Inherit via back propagation  datatype3=accumoutdatatype3  validOut=on  endInandOut=on  startOut=on  countOut=on  dim=-1  DoSatur=off  parallel=off
      settings: SourceProductBaseCode=SL
  Terminator : Terminator
  Terminator1 : Terminator
  Terminator2 : Terminator
  dataOut : Outport
  wires:
  Data Type Conversion/1 -> dataOut/1
  ? -> Terminator1/1  "validOut"
  In2/1 -> Multiply-Accumulate/1
  In3/1 -> ?
  Multiply-Accumulate/1 -> Data Type Conversion/1
  ? -> Terminator/1  "countOut"
  In1/1 -> Multiply-Accumulate/2
  ? -> Terminator2/1  "vectorOutValid"

== system model_cnn/HDL CNN Model/Dense Layer 1/Dense Layer 1/adder80 ==
  In1 : Inport
  In2 : Inport  Port=2
  In3 : Inport  Port=3
  Data Type Conversion : DataTypeConversion  OutDataTypeStr=datatypeLayer3
  Multiply-Accumulate : hdlsllib/HDL Operations/Multiply-Accumulate  opMode=Streaming - using Number of Samples  initValueSetting=Dialog  initValue=0  initValueSetting2=Dialog  initValue2=0  initValueSetting3=Dialog  initValue3=0  num_samples=1984  RndMeth2=Floor  RndMeth3=Floor  datatype2=Inherit: Inherit via back propagation  datatype3=accumoutdatatype3  validOut=on  endInandOut=on  startOut=on  countOut=on  dim=-1  DoSatur=off  parallel=off
      settings: SourceProductBaseCode=SL
  Terminator : Terminator
  Terminator1 : Terminator
  Terminator2 : Terminator
  dataOut : Outport
  wires:
  Data Type Conversion/1 -> dataOut/1
  ? -> Terminator1/1  "validOut"
  In2/1 -> Multiply-Accumulate/1
  In3/1 -> ?
  Multiply-Accumulate/1 -> Data Type Conversion/1
  ? -> Terminator/1  "countOut"
  In1/1 -> Multiply-Accumulate/2
  ? -> Terminator2/1  "vectorOutValid"

== system model_cnn/HDL CNN Model/Dense Layer 1/Dense Layer 1/adder81 ==
  In1 : Inport
  In2 : Inport  Port=2
  In3 : Inport  Port=3
  Data Type Conversion : DataTypeConversion  OutDataTypeStr=datatypeLayer3
  Multiply-Accumulate : hdlsllib/HDL Operations/Multiply-Accumulate  opMode=Streaming - using Number of Samples  initValueSetting=Dialog  initValue=0  initValueSetting2=Dialog  initValue2=0  initValueSetting3=Dialog  initValue3=0  num_samples=1984  RndMeth2=Floor  RndMeth3=Floor  datatype2=Inherit: Inherit via back propagation  datatype3=accumoutdatatype3  validOut=on  endInandOut=on  startOut=on  countOut=on  dim=-1  DoSatur=off  parallel=off
      settings: SourceProductBaseCode=SL
  Terminator : Terminator
  Terminator1 : Terminator
  Terminator2 : Terminator
  dataOut : Outport
  wires:
  Data Type Conversion/1 -> dataOut/1
  ? -> Terminator1/1  "validOut"
  In2/1 -> Multiply-Accumulate/1
  In3/1 -> ?
  Multiply-Accumulate/1 -> Data Type Conversion/1
  ? -> Terminator/1  "countOut"
  In1/1 -> Multiply-Accumulate/2
  ? -> Terminator2/1  "vectorOutValid"

== system model_cnn/HDL CNN Model/Dense Layer 1/Dense Layer 1/adder82 ==
  In1 : Inport
  In2 : Inport  Port=2
  In3 : Inport  Port=3
  Data Type Conversion : DataTypeConversion  OutDataTypeStr=datatypeLayer3
  Multiply-Accumulate : hdlsllib/HDL Operations/Multiply-Accumulate  opMode=Streaming - using Number of Samples  initValueSetting=Dialog  initValue=0  initValueSetting2=Dialog  initValue2=0  initValueSetting3=Dialog  initValue3=0  num_samples=1984  RndMeth2=Floor  RndMeth3=Floor  datatype2=Inherit: Inherit via back propagation  datatype3=accumoutdatatype3  validOut=on  endInandOut=on  startOut=on  countOut=on  dim=-1  DoSatur=off  parallel=off
      settings: SourceProductBaseCode=SL
  Terminator : Terminator
  Terminator1 : Terminator
  Terminator2 : Terminator
  dataOut : Outport
  wires:
  Data Type Conversion/1 -> dataOut/1
  ? -> Terminator1/1  "validOut"
  In2/1 -> Multiply-Accumulate/1
  In3/1 -> ?
  Multiply-Accumulate/1 -> Data Type Conversion/1
  ? -> Terminator/1  "countOut"
  In1/1 -> Multiply-Accumulate/2
  ? -> Terminator2/1  "vectorOutValid"

== system model_cnn/HDL CNN Model/Dense Layer 1/Dense Layer 1/adder83 ==
  In1 : Inport
  In2 : Inport  Port=2
  In3 : Inport  Port=3
  Data Type Conversion : DataTypeConversion  OutDataTypeStr=datatypeLayer3
  Multiply-Accumulate : hdlsllib/HDL Operations/Multiply-Accumulate  opMode=Streaming - using Number of Samples  initValueSetting=Dialog  initValue=0  initValueSetting2=Dialog  initValue2=0  initValueSetting3=Dialog  initValue3=0  num_samples=1984  RndMeth2=Floor  RndMeth3=Floor  datatype2=Inherit: Inherit via back propagation  datatype3=accumoutdatatype3  validOut=on  endInandOut=on  startOut=on  countOut=on  dim=-1  DoSatur=off  parallel=off
      settings: SourceProductBaseCode=SL
  Terminator : Terminator
  Terminator1 : Terminator
  Terminator2 : Terminator
  dataOut : Outport
  wires:
  Data Type Conversion/1 -> dataOut/1
  ? -> Terminator1/1  "validOut"
  In2/1 -> Multiply-Accumulate/1
  In3/1 -> ?
  Multiply-Accumulate/1 -> Data Type Conversion/1
  ? -> Terminator/1  "countOut"
  In1/1 -> Multiply-Accumulate/2
  ? -> Terminator2/1  "vectorOutValid"

== system model_cnn/HDL CNN Model/Dense Layer 1/Dense Layer 1/adder84 ==
  In1 : Inport
  In2 : Inport  Port=2
  In3 : Inport  Port=3
  Data Type Conversion : DataTypeConversion  OutDataTypeStr=datatypeLayer3
  Multiply-Accumulate : hdlsllib/HDL Operations/Multiply-Accumulate  opMode=Streaming - using Number of Samples  initValueSetting=Dialog  initValue=0  initValueSetting2=Dialog  initValue2=0  initValueSetting3=Dialog  initValue3=0  num_samples=1984  RndMeth2=Floor  RndMeth3=Floor  datatype2=Inherit: Inherit via back propagation  datatype3=accumoutdatatype3  validOut=on  endInandOut=on  startOut=on  countOut=on  dim=-1  DoSatur=off  parallel=off
      settings: SourceProductBaseCode=SL
  Terminator : Terminator
  Terminator1 : Terminator
  Terminator2 : Terminator
  dataOut : Outport
  wires:
  Data Type Conversion/1 -> dataOut/1
  ? -> Terminator1/1  "validOut"
  In2/1 -> Multiply-Accumulate/1
  In3/1 -> ?
  Multiply-Accumulate/1 -> Data Type Conversion/1
  ? -> Terminator/1  "countOut"
  In1/1 -> Multiply-Accumulate/2
  ? -> Terminator2/1  "vectorOutValid"

== system model_cnn/HDL CNN Model/Dense Layer 1/Dense Layer 1/adder85 ==
  In1 : Inport
  In2 : Inport  Port=2
  In3 : Inport  Port=3
  Data Type Conversion : DataTypeConversion  OutDataTypeStr=datatypeLayer3
  Multiply-Accumulate : hdlsllib/HDL Operations/Multiply-Accumulate  opMode=Streaming - using Number of Samples  initValueSetting=Dialog  initValue=0  initValueSetting2=Dialog  initValue2=0  initValueSetting3=Dialog  initValue3=0  num_samples=1984  RndMeth2=Floor  RndMeth3=Floor  datatype2=Inherit: Inherit via back propagation  datatype3=accumoutdatatype3  validOut=on  endInandOut=on  startOut=on  countOut=on  dim=-1  DoSatur=off  parallel=off
      settings: SourceProductBaseCode=SL
  Terminator : Terminator
  Terminator1 : Terminator
  Terminator2 : Terminator
  dataOut : Outport
  wires:
  Data Type Conversion/1 -> dataOut/1
  ? -> Terminator1/1  "validOut"
  In2/1 -> Multiply-Accumulate/1
  In3/1 -> ?
  Multiply-Accumulate/1 -> Data Type Conversion/1
  ? -> Terminator/1  "countOut"
  In1/1 -> Multiply-Accumulate/2
  ? -> Terminator2/1  "vectorOutValid"

== system model_cnn/HDL CNN Model/Dense Layer 1/Dense Layer 1/adder86 ==
  In1 : Inport
  In2 : Inport  Port=2
  In3 : Inport  Port=3
  Data Type Conversion : DataTypeConversion  OutDataTypeStr=datatypeLayer3
  Multiply-Accumulate : hdlsllib/HDL Operations/Multiply-Accumulate  opMode=Streaming - using Number of Samples  initValueSetting=Dialog  initValue=0  initValueSetting2=Dialog  initValue2=0  initValueSetting3=Dialog  initValue3=0  num_samples=1984  RndMeth2=Floor  RndMeth3=Floor  datatype2=Inherit: Inherit via back propagation  datatype3=accumoutdatatype3  validOut=on  endInandOut=on  startOut=on  countOut=on  dim=-1  DoSatur=off  parallel=off
      settings: SourceProductBaseCode=SL
  Terminator : Terminator
  Terminator1 : Terminator
  Terminator2 : Terminator
  dataOut : Outport
  wires:
  Data Type Conversion/1 -> dataOut/1
  ? -> Terminator1/1  "validOut"
  In2/1 -> Multiply-Accumulate/1
  In3/1 -> ?
  Multiply-Accumulate/1 -> Data Type Conversion/1
  ? -> Terminator/1  "countOut"
  In1/1 -> Multiply-Accumulate/2
  ? -> Terminator2/1  "vectorOutValid"

== system model_cnn/HDL CNN Model/Dense Layer 1/Dense Layer 1/adder87 ==
  In1 : Inport
  In2 : Inport  Port=2
  In3 : Inport  Port=3
  Data Type Conversion : DataTypeConversion  OutDataTypeStr=datatypeLayer3
  Multiply-Accumulate : hdlsllib/HDL Operations/Multiply-Accumulate  opMode=Streaming - using Number of Samples  initValueSetting=Dialog  initValue=0  initValueSetting2=Dialog  initValue2=0  initValueSetting3=Dialog  initValue3=0  num_samples=1984  RndMeth2=Floor  RndMeth3=Floor  datatype2=Inherit: Inherit via back propagation  datatype3=accumoutdatatype3  validOut=on  endInandOut=on  startOut=on  countOut=on  dim=-1  DoSatur=off  parallel=off
      settings: SourceProductBaseCode=SL
  Terminator : Terminator
  Terminator1 : Terminator
  Terminator2 : Terminator
  dataOut : Outport
  wires:
  Data Type Conversion/1 -> dataOut/1
  ? -> Terminator1/1  "validOut"
  In2/1 -> Multiply-Accumulate/1
  In3/1 -> ?
  Multiply-Accumulate/1 -> Data Type Conversion/1
  ? -> Terminator/1  "countOut"
  In1/1 -> Multiply-Accumulate/2
  ? -> Terminator2/1  "vectorOutValid"

== system model_cnn/HDL CNN Model/Dense Layer 1/Dense Layer 1/adder88 ==
  In1 : Inport
  In2 : Inport  Port=2
  In3 : Inport  Port=3
  Data Type Conversion : DataTypeConversion  OutDataTypeStr=datatypeLayer3
  Multiply-Accumulate : hdlsllib/HDL Operations/Multiply-Accumulate  opMode=Streaming - using Number of Samples  initValueSetting=Dialog  initValue=0  initValueSetting2=Dialog  initValue2=0  initValueSetting3=Dialog  initValue3=0  num_samples=1984  RndMeth2=Floor  RndMeth3=Floor  datatype2=Inherit: Inherit via back propagation  datatype3=accumoutdatatype3  validOut=on  endInandOut=on  startOut=on  countOut=on  dim=-1  DoSatur=off  parallel=off
      settings: SourceProductBaseCode=SL
  Terminator : Terminator
  Terminator1 : Terminator
  Terminator2 : Terminator
  dataOut : Outport
  wires:
  Data Type Conversion/1 -> dataOut/1
  ? -> Terminator1/1  "validOut"
  In2/1 -> Multiply-Accumulate/1
  In3/1 -> ?
  Multiply-Accumulate/1 -> Data Type Conversion/1
  ? -> Terminator/1  "countOut"
  In1/1 -> Multiply-Accumulate/2
  ? -> Terminator2/1  "vectorOutValid"

== system model_cnn/HDL CNN Model/Dense Layer 1/Dense Layer 1/adder89 ==
  In1 : Inport
  In2 : Inport  Port=2
  In3 : Inport  Port=3
  Data Type Conversion : DataTypeConversion  OutDataTypeStr=datatypeLayer3
  Multiply-Accumulate : hdlsllib/HDL Operations/Multiply-Accumulate  opMode=Streaming - using Number of Samples  initValueSetting=Dialog  initValue=0  initValueSetting2=Dialog  initValue2=0  initValueSetting3=Dialog  initValue3=0  num_samples=1984  RndMeth2=Floor  RndMeth3=Floor  datatype2=Inherit: Inherit via back propagation  datatype3=accumoutdatatype3  validOut=on  endInandOut=on  startOut=on  countOut=on  dim=-1  DoSatur=off  parallel=off
      settings: SourceProductBaseCode=SL
  Terminator : Terminator
  Terminator1 : Terminator
  Terminator2 : Terminator
  dataOut : Outport
  wires:
  Data Type Conversion/1 -> dataOut/1
  ? -> Terminator1/1  "validOut"
  In2/1 -> Multiply-Accumulate/1
  In3/1 -> ?
  Multiply-Accumulate/1 -> Data Type Conversion/1
  ? -> Terminator/1  "countOut"
  In1/1 -> Multiply-Accumulate/2
  ? -> Terminator2/1  "vectorOutValid"

== system model_cnn/HDL CNN Model/Dense Layer 1/Dense Layer 1/adder9 ==
  In1 : Inport
  In2 : Inport  Port=2
  In3 : Inport  Port=3
  Data Type Conversion : DataTypeConversion  OutDataTypeStr=datatypeLayer3
  Multiply-Accumulate : hdlsllib/HDL Operations/Multiply-Accumulate  opMode=Streaming - using Number of Samples  initValueSetting=Dialog  initValue=0  initValueSetting2=Dialog  initValue2=0  initValueSetting3=Dialog  initValue3=0  num_samples=1984  RndMeth2=Floor  RndMeth3=Floor  datatype2=Inherit: Inherit via back propagation  datatype3=accumoutdatatype3  validOut=on  endInandOut=on  startOut=on  countOut=on  dim=-1  DoSatur=off  parallel=off
      settings: SourceProductBaseCode=SL
  Terminator : Terminator
  Terminator1 : Terminator
  Terminator2 : Terminator
  dataOut : Outport
  wires:
  Data Type Conversion/1 -> dataOut/1
  ? -> Terminator1/1  "validOut"
  In2/1 -> Multiply-Accumulate/1
  In3/1 -> ?
  Multiply-Accumulate/1 -> Data Type Conversion/1
  ? -> Terminator/1  "countOut"
  In1/1 -> Multiply-Accumulate/2
  ? -> Terminator2/1  "vectorOutValid"
